simulink model "MCP_rotation_pressureOLub"  (R2020a)
settings: configuration reference "globalConfig" (kept outside this file)
undefined symbols (not defined in the file): A, B, C, D, magnitude
libraries: simulink_extras x1, cstblocks x1
settings Model: Creator=victo  LastModifiedBy=victo
settings ConfigSetRef: SourceName=globalConfig  SourceLocation=Base Workspace

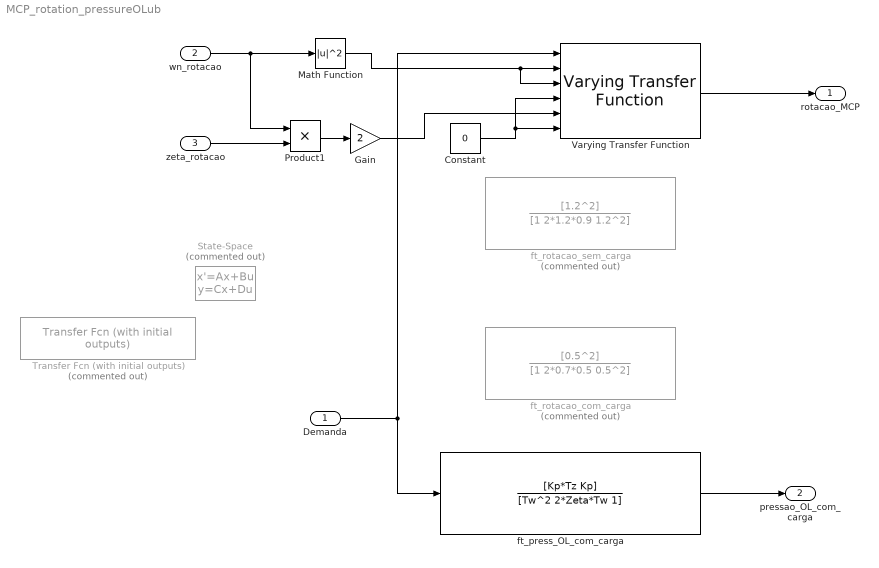
== system MCP_rotation_pressureOLub ==
  Demanda : Inport  OutDataTypeStr=double  PortDimensions=1  SampleTime=0
  wn_rotacao : Inport  Port=2
  zeta_rotacao : Inport  Port=3
  Constant : Constant  Value=0
  Gain : Gain  Gain=2
  Math Function : Math  Operator=magnitude^2  SaturateOnIntegerOverflow=on
  Product1 : Product
  State-Space : StateSpace  Commented=on  A=A  B=B  C=C  D=D  InitialCondition=600
  Transfer Fcn (with initial outputs) : simulink_extras/Additional Linear/Transfer Fcn (with initial outputs)  Commented=on  N=[0.0548 0.0518]  D=[1 1.541 0.1773]  Y0=600  U0=600
  Varying Transfer Function : cstblocks/Linear Parameter Varying/Varying Transfer Function  N=2
  ft_press_OL_com_carga : TransferFcn  Numerator=[Kp*Tz Kp]  Denominator=[Tw^2 2*Zeta*Tw 1]  mask{Kp=0.34722, Tz=13.563, Tw=7.2155, Zeta=0.97827, Td=0}
  ft_rotacao_com_carga : TransferFcn  Commented=on  Numerator=[0.5^2]  Denominator=[1 2*0.7*0.5 0.5^2]
  ft_rotacao_sem_carga : TransferFcn  Commented=on  Numerator=[1.2^2]  Denominator=[1 2*1.2*0.9 1.2^2]
  rotacao_MCP : Outport
  pressao_OL_com_carga : Outport  Port=2  OutDataTypeStr=double  PortDimensions=1  SampleTime=0
  wires:
  Demanda/1 -> Varying Transfer Function/1, ft_press_OL_com_carga/1
  ft_press_OL_com_carga/1 -> pressao_OL_com_carga/1
  Varying Transfer Function/1 -> rotacao_MCP/1
  Constant/1 -> Varying Transfer Function/4, Varying Transfer Function/6
  Gain/1 -> Varying Transfer Function/5
  Math Function/1 -> Varying Transfer Function/3, Varying Transfer Function/2
  wn_rotacao/1 -> Product1/1, Math Function/1
  zeta_rotacao/1 -> Product1/2
  Product1/1 -> Gain/1
